simulink model "VSMRAC"  (R2018a)
settings: Solver=ode45  StartTime=0.0  StopTime=10  RelTol=1e-3  EnableMultiTasking=on
InitFcn:
  | u = 0;
  | ym = 0;
  | y = 0.5;
  | eo = 0;
  | am = 1;
  | km = 1;
  | ap = -1.1;
  | kp = 1;
  | theta1 = 2;
  | theta2 = 1;
  | theta1_estimated = 2.3;
  | theta2_estimated = 1.3;
  | sigma = 0.9;
settings Model: Creator=danilopena  LastModifiedBy=LIME
settings DataIOCC: LimitDataPoints=on  SaveFormat=Array
settings OptimizationCC: LifeSpan=inf
settings DebuggingCC: UnderspecifiedInitializationDetection=Classic  MergeDetectMultiDrivingBlocksExec=none  SolverPrmCheckMsg=warning  StateNameClashWarn=warning  SFUnexpectedBacktrackingDiag=warning  SFNoUnconditionalDefaultTransitionDiag=warning  SFExecutionAtInitializationDiag=none
settings HardwareCC: ProdBitPerPointer=32  ProdBitPerSizeT=32  ProdBitPerPtrDiffT=32  ProdLargestAtomicFloat=None  ProdIntDivRoundTo=Undefined  ProdEndianess=Unspecified  ProdWordSize=32  ProdHWDeviceType=32-bit Generic
settings ModelReferenceCC: PropagateSignalLabelsOutOfModel=off
settings CodeAppCC: StateflowObjectComments=on
settings GRTTargetCC: TargetLangStandard=C89/C90 (ANSI)  GeneratePreprocessorConditionals=Disable all
settings ConfigComp: CovMetricSettings=dw  CovHtmlReporting=on  CovSaveCumulativeToWorkspaceVar=on  CovSaveSingleToWorkspaceVar=on  CovExternalEMLEnable=off

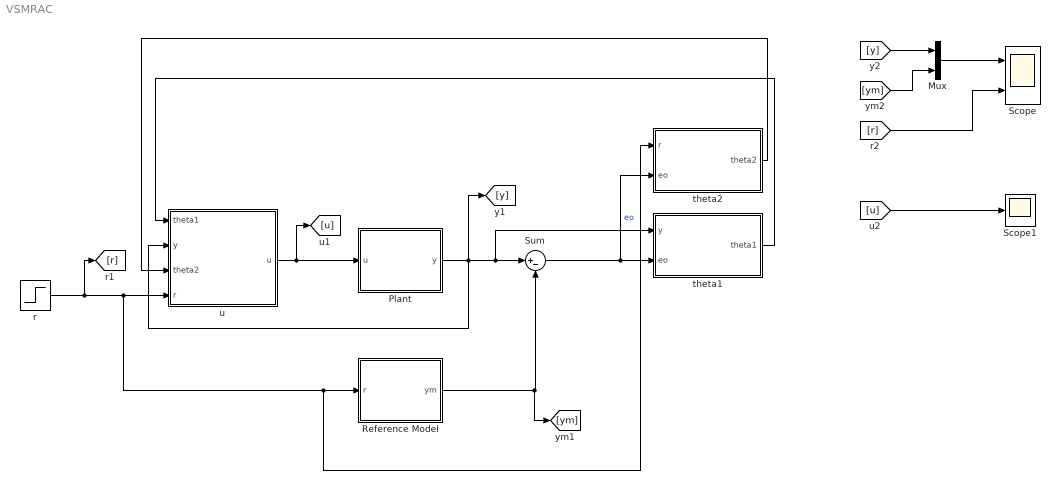
== system VSMRAC ==
  Mux : Mux  Inputs=2
  Plant : Subsystem
  Reference Model : Subsystem
  Scope : Scope  NumInputPorts=2
  Scope1 : Scope
  Sum : Sum  Inputs=|+-
  r : Step  SampleTime=0
  theta1 : Subsystem
  theta2 : Subsystem
  u : Subsystem
  wires:
  Plant/1(y) -> [y], u/2(y), theta1/1(y), Sum/1
  Reference Model/1(ym) -> [ym], Sum/2
  Sum/1 -> theta2/2(eo), theta1/2(eo)  "eo"
  u/1(u) -> [u], Plant/1(u)
  theta1/1(theta1) -> u/1(theta1)
  theta2/1(theta2) -> u/3(theta2)
  r/1 -> [r], theta2/1(r), Reference Model/1(r), u/4(r)
  [r] -> Scope/2
  [y] -> Mux/1
  [ym] -> Mux/2
  Mux/1 -> Scope/1
  [u] -> Scope1/1

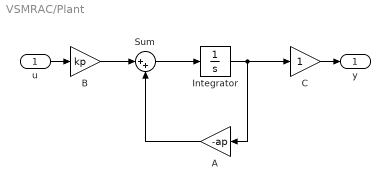
== system VSMRAC/Plant ==
  u : Inport
  A : Gain  Gain=-ap
  B : Gain  Gain=kp
  C : Gain
  Integrator : Integrator
  Sum : Sum  Inputs=|++
  y : Outport
  wires:
  B/1 -> Sum/1
  A/1 -> Sum/2
  Sum/1 -> Integrator/1
  Integrator/1 -> C/1, A/1
  u/1 -> B/1
  C/1 -> y/1

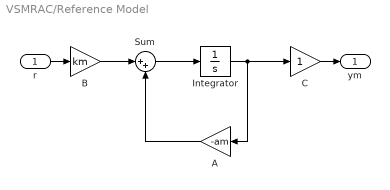
== system VSMRAC/Reference Model ==
  r : Inport
  A : Gain  Gain=-am
  B : Gain  Gain=km
  C : Gain
  Integrator : Integrator
  Sum : Sum  Inputs=|++
  ym : Outport
  wires:
  B/1 -> Sum/1
  A/1 -> Sum/2
  Sum/1 -> Integrator/1
  Integrator/1 -> C/1, A/1
  r/1 -> B/1
  C/1 -> ym/1

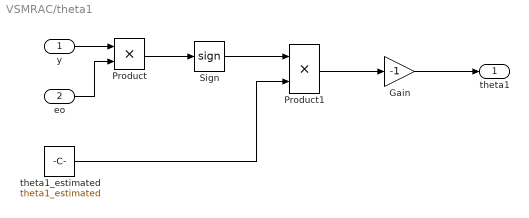
== system VSMRAC/theta1 ==
  y : Inport
  eo : Inport  Port=2
  Gain : Gain  Gain=-1
  Product : Product
  Product1 : Product
  Sign : Signum  ZeroCross=off
  theta1_estimated : Constant  Value=theta1_estimated
  theta1 : Outport
  wires:
  y/1 -> Product/1
  eo/1 -> Product/2
  Product/1 -> Sign/1
  Sign/1 -> Product1/1
  theta1_estimated/1 -> Product1/2
  Product1/1 -> Gain/1
  Gain/1 -> theta1/1

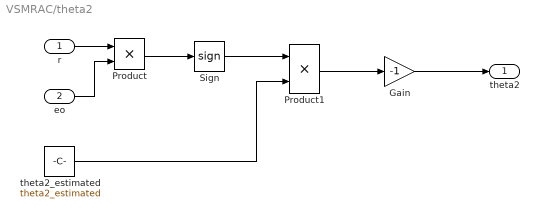
== system VSMRAC/theta2 ==
  r : Inport
  eo : Inport  Port=2
  Gain : Gain  Gain=-1
  Product : Product
  Product1 : Product
  Sign : Signum  ZeroCross=off
  theta2_estimated : Constant  Value=theta2_estimated
  theta2 : Outport
  wires:
  r/1 -> Product/1
  eo/1 -> Product/2
  Product/1 -> Sign/1
  Sign/1 -> Product1/1
  theta2_estimated/1 -> Product1/2
  Product1/1 -> Gain/1
  Gain/1 -> theta2/1

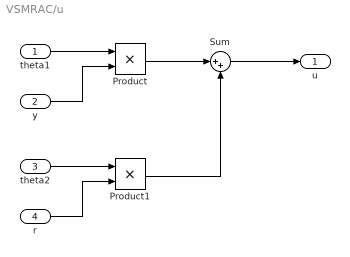
== system VSMRAC/u ==
  theta1 : Inport
  y : Inport  Port=2
  theta2 : Inport  Port=3
  r : Inport  Port=4
  Product : Product
  Product1 : Product
  Sum : Sum  Inputs=|++
  u : Outport
  wires:
  y/1 -> Product/2
  theta1/1 -> Product/1
  r/1 -> Product1/2
  theta2/1 -> Product1/1
  Product/1 -> Sum/1
  Product1/1 -> Sum/2
  Sum/1 -> u/1
